simulink model "simu"  (R2024b)
settings: Solver=VariableStepAuto  StartTime=0.0  StopTime=0.01  RelTol=1e-3
values from neighbouring files (symbols this model uses):
  C = 0.00001    (= 1e-05)    [odeBUck.m]
  L = 0.002    [odeBUck.m]
  R = 10    [odeBUck.m]
  Uin = 32    [odeBUck.m]
settings Model: Creator=USER
settings RTWCC: GPUComputeCapability=3.5

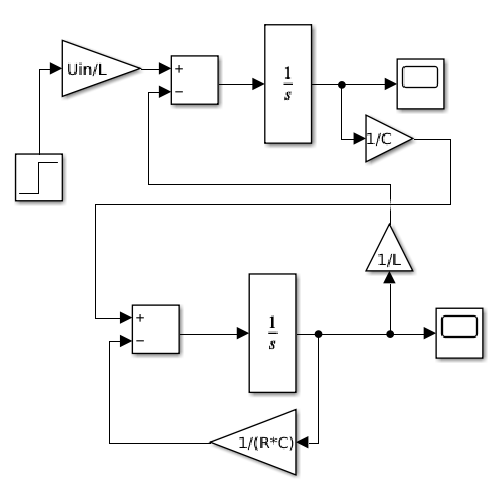
[thumbnail: Simulink's stored preview of the top-level diagram]
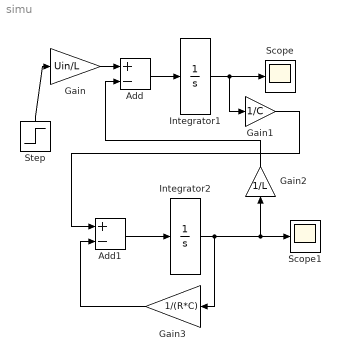
== system simu ==
  Add : Sum  Inputs=+-
  Add1 : Sum  Inputs=+-
  Gain : Gain  Gain=Uin/L
  Gain1 : Gain  Gain=1/C
  Gain2 : Gain  Gain=1/L
  Gain3 : Gain  Gain=1/(R*C)
  Integrator1 : Integrator
  Integrator2 : Integrator
  Scope : Scope
  Scope1 : Scope
  Step : Step  Time=0  SampleTime=0
  wires:
  Add1/1 -> Integrator2/1
  Gain1/1 -> Add1/1
  Gain2/1 -> Add/2
  Integrator1/1 -> Scope/1, Gain1/1
  Integrator2/1 -> Gain3/1, Scope1/1, Gain2/1
  Step/1 -> Gain/1
  Gain/1 -> Add/1
  Add/1 -> Integrator1/1
  Gain3/1 -> Add1/2
